simulink model "flatball_6dof"  (R2021b)
settings: Solver=ode1be  StartTime=0.0  StopTime=30  FixedStep=1e-3  MaxStep=0.01  MinStep=0.01  RelTol=1e-3
values from neighbouring files (symbols this model uses):
  amb = evalin( 'base', 'amb')    [flatball_6dof_eqom.m]
  C = evalin( 'base', 'C')    [flatball_6dof_eqom.m]
  disc = evalin( 'base', 'disc')    [flatball_6dof_eqom.m]    (also in flatball_6dof_init.m = struct; flatball_init_disc_params.m = struct)
  X0_z1m_at_rest = [1e-3 1e-3 -1, -1e-6 1e-6 -1e-6, 0 0 1e-6, 0 0 -1e-6]    [flatball_6dof_wrk.m]    (also in hummel_thesis_mdl_validation.m)
undefined symbols (not defined in the file or in its folder): clock, flatball, flatball_6dof_plnt_lib, HandH
libraries: simulink x6, aerolibanim x3, aerolibnav x3, matrix_library x3, mspfiltlib x1, hucker_lib x1
(part 1 of 3)
settings Model: Creator=misc.protolabs@gmail.com  LastModifiedBy=schae
settings SolverCC: InitialStep=0.01  NumberNewtonIterations=10
settings DataIOCC: SaveFormat=StructureWithTime  SaveOutput=off  DSMLogging=off  SaveTime=off  ReturnWorkspaceOutputsName=simout
settings DebuggingCC: InheritedTsInSrcMsg=none

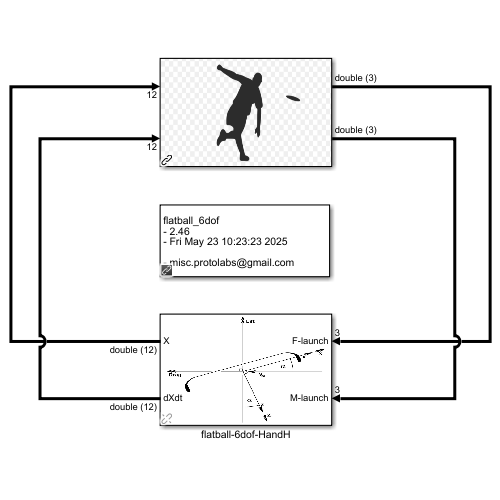
[thumbnail: Simulink's stored preview of the top-level diagram]
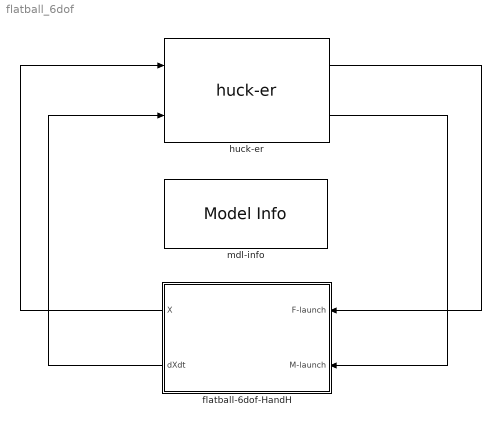
== system flatball_6dof ==
  flatball-6dof-HandH : Subsystem  AncestorBlock=flatball_6dof_plnt_lib/flatball-6dof-HandH
      mask Display: image('C:\.local\desktop\misc.protolabs\flatball-aero-ssl\arxiv\img\screenshots\flatball-6dof.png'); % Use "Edit Image" on toolstrip to change.
  huck-er : hucker_lib/huck-er  SystemSampleTime=-1  VariantActivationTime=update diagram  Latency=0  AutoFrameSizeCalculation=off
      mask Display: image('C:\.local\desktop\misc.protolabs\flatball-aero-ssl\arxiv\img\screenshots\hucker.png'); % Use "Edit Image" on toolstrip to change.
  mdl-info : simulink/Model-Wide Utilities/Model Info  Frame=on  DisplayStringWithTags=|  HorizontalTextAlignment=Left  LeftAlignmentValue=0.02
      | flatball_6dof
      | - %<ModelVersion>
      | - %<LastModificationDate>
      | 
      | - %<Creator>
  wires:
  flatball-6dof-HandH/2(dXdt) -> huck-er/2
  flatball-6dof-HandH/1(X) -> huck-er/1
  huck-er/1 -> flatball-6dof-HandH/1(F-launch)
  huck-er/2 -> flatball-6dof-HandH/2(M-launch)

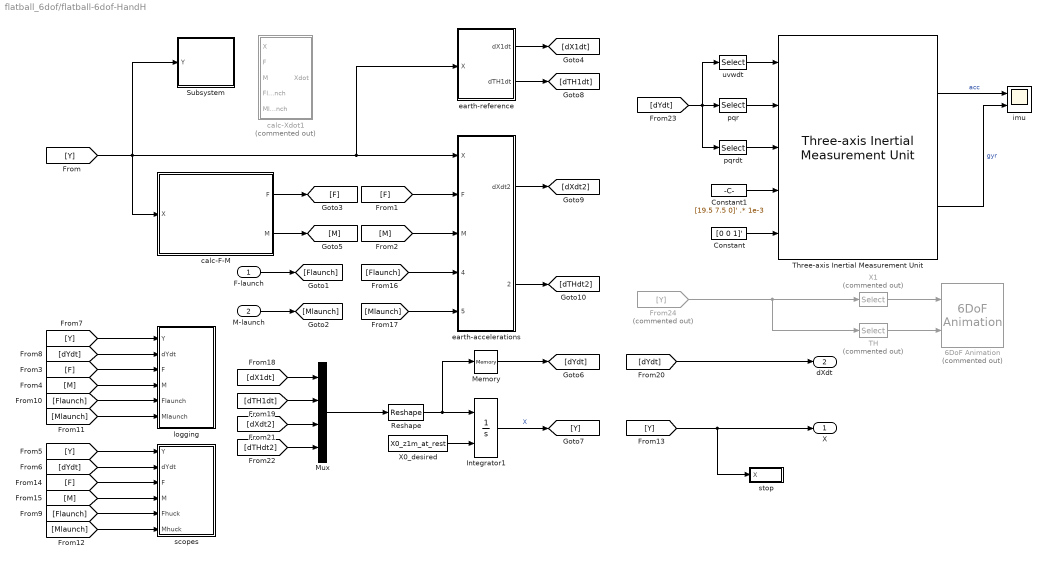
== system flatball_6dof/flatball-6dof-HandH ==
  F-launch : Inport
  M-launch : Inport  Port=2
  6DoF Animation : aerolibanim/6DoF Animation  Commented=on  u1=[0 50 -20 20 -5 0]  u2=0.01  u3=1.0  u4=[50 0 0]  u5=Fixed position  u6=[150 150 25]  u7=10  u8=on
  Constant : Constant  Value=[0 0 1]'
  Constant1 : Constant  Value=[19.5 7.5 0]' .* 1e-3
  From24 : From  Commented=on  GotoTag=Y
  Integrator1 : Integrator  InitialConditionSource=external
  Memory : Memory
  Mux : Mux
  Reshape : Reshape
  Subsystem : Subsystem
  TH : Selector  Commented=on  InputPortWidth=12  IndexOptions=Index vector (dialog)  Indices=[4 5 6]  OutputSizes=1
  Three-axis Inertial Measurement Unit : aerolibnav/Three-axis Inertial Measurement Unit  units=Metric (MKS)  imu=[0 0 0]  i_Ts=0.01  dtype_a=on  w_a=2*pi*50  z_a=0.707  a_sf_cc=[1 0 0; 0 1 0; 0 0 1]  a_bias=[0 0 0]  a_sat=[-1 -1 -1 1 1 1] .* 16*amb.g  dtype_g=on  w_g=2*pi*50  z_g=0.707  g_sf_cc=[1 0 0; 0 1 0; 0 0 1]  g_bias=[0 0 0]  g_sens=[0 0 0]  g_sat=[-1 -1 -1 1 1 1] .* 4000*C.DEG2RAD  i_rand=on  i_seeds=ceil( round( clock, 1))  i_pow=[1 1 1 0.1 0.1 0.1] .* 1e-4
  X0_desired : Constant  Value=X0_z1m_at_rest
  X1 : Selector  Commented=on  InputPortWidth=12  IndexOptions=Index vector (dialog)  Indices=[1 2 3]  OutputSizes=1
  calc-F-M : Subsystem
  calc-Xdot1 : Subsystem  Commented=on
  earth-accelerations : Subsystem
  earth-reference : Subsystem
  imu : Scope  NumInputPorts=2
  logging : Subsystem
  pqr : Selector  InputPortWidth=12  IndexOptions=Index vector (dialog)  Indices=[4 5 6]  OutputSizes=1
  pqrdt : Selector  InputPortWidth=12  IndexOptions=Index vector (dialog)  Indices=[10 11 12]  OutputSizes=1
  scopes : Subsystem
  stop : Subsystem
  uvwdt : Selector  InputPortWidth=12  IndexOptions=Index vector (dialog)  Indices=[7 8 9]  OutputSizes=1
  X : Outport
  dXdt : Outport  Port=2
  wires:
  [Flaunch] -> scopes/5(Fhuck)
  [M] -> scopes/4(M)
  [F] -> scopes/3(F)
  [M] -> logging/4(M)
  [Mlaunch] -> logging/6(Mlaunch)
  [Flaunch] -> logging/5(Flaunch)
  [Mlaunch] -> scopes/6(Mhuck)
  [F] -> logging/3(F)
  [Y] -> scopes/1(Y)
  [dYdt] -> scopes/2(dYdt)
  [dYdt] -> logging/2(dYdt)
  [Y] -> logging/1(Y)
  [Y] -> stop/1(X), X/1
  F-launch/1 -> [Flaunch]
  M-launch/1 -> [Mlaunch]
  [Y] -> earth-reference/1(X), earth-accelerations/1(X), Subsystem/1(Y), calc-F-M/1(X)
  [M] -> earth-accelerations/3(M)
  X0_desired/1 -> Integrator1/2
  [F] -> earth-accelerations/2(F)
  calc-F-M/2(M) -> [M]
  calc-F-M/1(F) -> [F]
  Integrator1/1 -> [Y]  "X"
  [Flaunch] -> earth-accelerations/4(Flaunch)
  [Mlaunch] -> earth-accelerations/5(Mlaunch)
  Memory/1 -> [dYdt]
  earth-reference/1(dX1dt) -> [dX1dt]
  earth-reference/2(dTH1dt) -> [dTH1dt]
  earth-accelerations/1(dXdt2) -> [dXdt2]
  earth-accelerations/2(dTHdt2) -> [dTHdt2]
  [dTHdt2] -> Mux/4
  [dXdt2] -> Mux/3
  [dTH1dt] -> Mux/2
  [dX1dt] -> Mux/1
  Mux/1 -> Reshape/1
  [dYdt] -> dXdt/1
  Reshape/1 -> Memory/1, Integrator1/1
  [dYdt] -> uvwdt/1, pqrdt/1, pqr/1
  pqr/1 -> Three-axis Inertial Measurement Unit/2
  Constant/1 -> Three-axis Inertial Measurement Unit/5
  Constant1/1 -> Three-axis Inertial Measurement Unit/4
  pqrdt/1 -> Three-axis Inertial Measurement Unit/3
  uvwdt/1 -> Three-axis Inertial Measurement Unit/1
  Three-axis Inertial Measurement Unit/1 -> imu/1  "acc"
  Three-axis Inertial Measurement Unit/2 -> imu/2  "gyr"
  From24/1 -> TH/1, X1/1
  TH/1 -> 6DoF Animation/2
  X1/1 -> 6DoF Animation/1

== system flatball_6dof/flatball-6dof-HandH/Subsystem ==
  Y : Inport
  Product : Product  Multiplication=Matrix(*)
  Scope : Scope  NumInputPorts=2
  TH : Selector  InputPortWidth=12  IndexOptions=Index vector (dialog)  Indices=[4 5 6]  OutputSizes=1
  TH1 : Selector  InputPortWidth=3  IndexOptions=Index vector (dialog)  Indices=[1 2]  OutputSizes=1
  TH2 : Selector  InputPortWidth=3  IndexOptions=Index vector (dialog)  Indices=[1 2]  OutputSizes=1
  Terminator : Terminator
  Transpose : Math  Operator=transpose  SaturateOnIntegerOverflow=on
  attitude-transform : MATLAB Function  TreatAsAtomicUnit=on
  rate-transform : MATLAB Function  TreatAsAtomicUnit=on
  wires:
  TH/1 -> Product/2, TH1/1, rate-transform/1(TH), attitude-transform/1(TH)
  rate-transform/1(T) -> [Tr21]
  attitude-transform/1(T) -> [Ta21]
  Y/1 -> TH/1
  [Tr21] -> Terminator/1
  [Ta21] -> Transpose/1
  Transpose/1 -> Product/1
  Product/1 -> TH2/1  "TH2"
  TH1/1 -> Scope/1
  TH2/1 -> Scope/2

== system flatball_6dof/flatball-6dof-HandH/calc-F-M ==
  X : Inport
  From1 : From  Commented=on  GotoTag=X
  From10 : From  Commented=on  GotoTag=F
  From11 : From  Commented=on  GotoTag=M
  From5 : From  Commented=on  GotoTag=alpha
  From6 : From  Commented=on  GotoTag=T
  From9 : From  Commented=on  GotoTag=wD
  TH : Selector  InputPortWidth=12  IndexOptions=Index vector (dialog)  Indices=[4 5 6]  OutputSizes=1
  T_c_N : MATLAB Function  TreatAsAtomicUnit=on
  calc-F : Subsystem
  calc-M : Subsystem
  calc-alpha : Subsystem
  lab : Subsystem  Commented=on
  F : Outport
  M : Outport  Port=2
  wires:
  From1/1 -> lab/1(X)
  From10/1 -> lab/5(F)
  From6/1 -> lab/2(T)
  X/1 -> TH/1, calc-M/1(X), calc-alpha/1(X), calc-F/1(X)
  [T] -> calc-M/2(T_c_N), calc-F/2(T_c_N)
  From9/1 -> lab/3(wD)
  [T] -> calc-alpha/2(T_c_N)
  [alpha] -> calc-F/3(alpha), calc-M/3(alpha)
  From11/1 -> lab/6(M)
  calc-alpha/1(alpha) -> [alpha]
  From5/1 -> lab/4(alpha)
  calc-F/1(F) -> F/1  "F2"
  calc-M/1(M) -> M/1  "M2"
  TH/1 -> T_c_N/1(TH)
  T_c_N/1(T_c_N) -> [T]

== system flatball_6dof/flatball-6dof-HandH/calc-Xdot1 ==
  X : Inport
  F : Inport  Port=2
  M : Inport  Port=3
  Flaunch : Inport  Port=4
  Mlaunch : Inport  Port=5
  Mux{,1..3} (4 alike) : Mux  Inputs=2
  Product1 : Product  Inputs=*/
  Reshape : Reshape
  Reshape1 : Reshape
  Reshape2 : Reshape
  Scope : Scope
  Scope1 : Scope
  Scope2 : Scope
  Selector : Selector  InputPortWidth=12  IndexOptions=Index vector (dialog)  Indices=[1 2 3 7 8 9 4 5 6 10 11 12]  OutputSizes=1
  Sum : Sum  Inputs=2
  calc-THdot : MATLAB Function  TreatAsAtomicUnit=on
  calc-Xdot : MATLAB Function  TreatAsAtomicUnit=on
  dTHdt : Selector  InputPortWidth=12  IndexOptions=Index vector (dialog)  Indices=[10 11 12]  OutputSizes=1
  dXdt : Selector  InputPortWidth=12  IndexOptions=Index vector (dialog)  Indices=[7 8 9]  OutputSizes=1
  mg : Constant  Value=disc.m
  Xdot : Outport
  wires:
  Reshape/1 -> Mux3/2
  Mux2/1 -> Mux/2
  Reshape1/1 -> Mux2/2
  dTHdt/1 -> Mux2/1
  dXdt/1 -> Mux1/1, calc-Xdot/1(dXdt), Mux3/1
  Reshape2/1 -> Sum/1
  Mux1/1 -> Scope/1, Mux/1
  calc-Xdot/1(Xdot) -> Reshape/1  "Xdot"
  calc-THdot/1(dTHdt2) -> Reshape1/1  "THdot"
  Product1/1 -> Mux1/2
  Sum/1 -> Product1/1, Scope2/1
  mg/1 -> Product1/2
  Flaunch/1 -> Sum/2, calc-Xdot/3(Flaunch)
  F/1 -> calc-Xdot/2(F), Reshape2/1
  Mlaunch/1 -> calc-THdot/3(Mlaunch)
  Selector/1 -> Xdot/1
  M/1 -> calc-THdot/2(M)
  X/1 -> calc-THdot/1(X), dXdt/1, dTHdt/1
  Mux/1 -> Selector/1

== system flatball_6dof/flatball-6dof-HandH/earth-accelerations ==
  X : Inport
  F : Inport  Port=2
  M : Inport  Port=3
  Flaunch : Inport  Port=4
  Mlaunch : Inport  Port=5
  Product1 : Product  Inputs=*/
  Sum : Sum  Inputs=2
  Sum1 : Sum  Inputs=2
  calc-THdot : MATLAB Function  TreatAsAtomicUnit=on
  mg : Constant  Value=disc.m
  dXdt2 : Outport
  dTHdt2 : Outport  Port=2
  wires:
  X/1 -> calc-THdot/1(X)
  Flaunch/1 -> Sum/2
  mg/1 -> Product1/2
  Sum/1 -> Product1/1
  Product1/1 -> dXdt2/1
  calc-THdot/1(dTHdt2) -> dTHdt2/1  "THdot"
  F/1 -> Sum/1
  Mlaunch/1 -> Sum1/2
  M/1 -> Sum1/1
  Sum1/1 -> calc-THdot/2(M)

== system flatball_6dof/flatball-6dof-HandH/earth-reference ==
  X : Inport
  dTHdt : Selector  InputPortWidth=12  IndexOptions=Index vector (dialog)  Indices=[10 11 12]  OutputSizes=1
  dXdt : Selector  InputPortWidth=12  IndexOptions=Index vector (dialog)  Indices=[7 8 9]  OutputSizes=1
  dX1dt : Outport
  dTH1dt : Outport  Port=2
  wires:
  X/1 -> dXdt/1, dTHdt/1
  dTHdt/1 -> dTH1dt/1
  dXdt/1 -> dX1dt/1

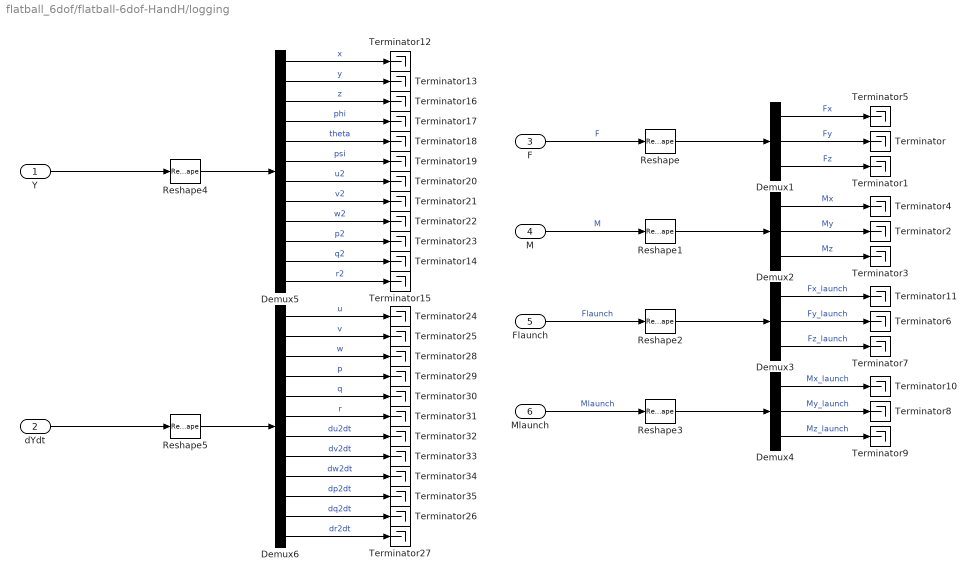
== system flatball_6dof/flatball-6dof-HandH/logging ==
  Y : Inport
  dYdt : Inport  Port=2
  F : Inport  Port=3
  M : Inport  Port=4
  Flaunch : Inport  Port=5
  Mlaunch : Inport  Port=6
  Demux{1..4} (4 alike) : Demux  Outputs=3
  Demux5 : Demux  Outputs=[1 1 1 1 1 1 1 1 1 1 1 1]
  Demux6 : Demux  Outputs=[1 1 1 1 1 1 1 1 1 1 1 1]
  Reshape{,1..5} (6 alike) : Reshape
  Terminator{,1..35} (36 alike) : Terminator
  wires:
  Reshape1/1 -> Demux2/1
  Demux2/3 -> Terminator3/1  "Mz"
  Demux2/1 -> Terminator4/1  "Mx"
  Reshape2/1 -> Demux3/1
  Demux1/3 -> Terminator1/1  "Fz"
  Demux1/2 -> Terminator/1  "Fy"
  Demux2/2 -> Terminator2/1  "My"
  Demux3/3 -> Terminator7/1  "Fz_launch"
  M/1 -> Reshape1/1  "M"
  Demux4/2 -> Terminator8/1  "My_launch"
  Demux1/1 -> Terminator5/1  "Fx"
  Reshape/1 -> Demux1/1
  Demux4/1 -> Terminator10/1  "Mx_launch"
  Demux4/3 -> Terminator9/1  "Mz_launch"
  Reshape3/1 -> Demux4/1
  Flaunch/1 -> Reshape2/1  "Flaunch"
  Demux3/1 -> Terminator11/1  "Fx_launch"
  Demux3/2 -> Terminator6/1  "Fy_launch"
  F/1 -> Reshape/1  "F"
  Mlaunch/1 -> Reshape3/1  "Mlaunch"
  Demux5/3 -> Terminator16/1  "z"
  Demux5/1 -> Terminator12/1  "x"
  Demux5/8 -> Terminator21/1  "v2"
  Demux5/9 -> Terminator22/1  "w2"
  Reshape4/1 -> Demux5/1
  Demux5/2 -> Terminator13/1  "y"
  Demux5/12 -> Terminator15/1  "r2"
  Demux5/10 -> Terminator23/1  "p2"
  Demux5/7 -> Terminator20/1  "u2"
  Demux5/5 -> Terminator18/1  "theta"
  Demux5/6 -> Terminator19/1  "psi"
  Demux5/11 -> Terminator14/1  "q2"
  Demux5/4 -> Terminator17/1  "phi"
  Y/1 -> Reshape4/1
  dYdt/1 -> Reshape5/1
  Demux6/4 -> Terminator29/1  "p"
  Demux6/11 -> Terminator26/1  "dq2dt"
  Demux6/6 -> Terminator31/1  "r"
  Demux6/5 -> Terminator30/1  "q"
  Demux6/7 -> Terminator32/1  "du2dt"
  Demux6/10 -> Terminator35/1  "dp2dt"
  Demux6/12 -> Terminator27/1  "dr2dt"
  Demux6/2 -> Terminator25/1  "v"
  Reshape5/1 -> Demux6/1
  Demux6/9 -> Terminator34/1  "dw2dt"
  Demux6/8 -> Terminator33/1  "dv2dt"
  Demux6/1 -> Terminator24/1  "u"
  Demux6/3 -> Terminator28/1  "w"

== system flatball_6dof/flatball-6dof-HandH/scopes ==
  Y : Inport
  dYdt : Inport  Port=2
  F : Inport  Port=3
  M : Inport  Port=4
  Fhuck : Inport  Port=5
  Mhuck : Inport  Port=6
  Compare To Constant : simulink/Logic and Bit Operations/Compare To Constant  relop=>=  const=0.0  OutDataTypeStr=boolean
  Demux : Demux  Outputs=[3 3 3 3]
  Demux1 : Demux  Outputs=[3 3 3 3]
  Selector : Selector  InputPortWidth=3  IndexOptions=Index vector (dialog)  Indices=[3]  OutputSizes=1
  Selector1 : Selector  InputPortWidth=3  IndexOptions=Index vector (dialog)  Indices=[1 2]  OutputSizes=1
  Stop Simulation : Stop
  Sum1 : Sum
  Sum2 : Sum
  TH1 : Scope
  TH1dot : Scope
  TH2dot : Scope
  TH2dotdot : Scope
  X1 : Scope
  X1dot : Scope
  X2dot : Scope
  X2dotdot : Scope
  eml-6dof : Subsystem  Commented=on
  flatball-F,M : Scope  NumInputPorts=2
  huck-F,M : Scope  NumInputPorts=2
  net-F,M : Scope  NumInputPorts=2
  work-in-progress : Subsystem  Commented=on
  wires:
  Sum2/1 -> net-F,M/2
  Mhuck/1 -> Sum2/2, huck-F,M/2
  Sum1/1 -> net-F,M/1
  Fhuck/1 -> Sum1/2, huck-F,M/1
  F/1 -> Sum1/1, flatball-F,M/1
  M/1 -> Sum2/1, flatball-F,M/2
  Demux/4 -> TH2dot/1
  dYdt/1 -> Demux1/1
  Selector/1 -> Compare To Constant/1
  Demux1/2 -> TH1dot/1
  Demux/2 -> Selector1/1
  Selector1/1 -> TH1/1
  Demux1/1 -> X1dot/1
  Demux/3 -> X2dot/1
  Demux1/4 -> TH2dotdot/1
  Compare To Constant/1 -> Stop Simulation/1
  Y/1 -> Demux/1
  Demux1/3 -> X2dotdot/1
  Demux/1 -> X1/1, Selector/1

== system flatball_6dof/flatball-6dof-HandH/stop ==
  X : Inport
  Compare To Constant : simulink/Logic and Bit Operations/Compare To Constant  relop=>=  const=0  OutDataTypeStr=boolean
  Selector : Selector  InputPortWidth=12  IndexOptions=Index vector (dialog)  Indices=[3]  OutputSizes=1
  Stop Simulation : Stop
  wires:
  Selector/1 -> Compare To Constant/1
  Compare To Constant/1 -> Stop Simulation/1
  X/1 -> Selector/1

== system flatball_6dof/flatball-6dof-HandH/calc-F-M/calc-F ==
  X : Inport
  T_c_N : Inport  Port=2
  alpha : Inport  Port=3
  Fg_N : Constant  Value=[0 0 disc.m*amb.g]'
  Terminator{,1..3} (4 alike) : Terminator
  aero-coeff : Subsystem
  calc-F : MATLAB Function  TreatAsAtomicUnit=on
  dXdt : Selector  InputPortWidth=12  IndexOptions=Index vector (dialog)  Indices=[7 8 9]  OutputSizes=1
  q-inf : Subsystem
  F : Outport
  wires:
  dXdt/1 -> calc-F/1(vel)
  X/1 -> dXdt/1, q-inf/1(X)
  T_c_N/1 -> calc-F/2(T_c_N)
  Fg_N/1 -> calc-F/3(Fg_N)
  calc-F/1(F) -> F/1  "F"
  q-inf/1(q-inf-S) -> calc-F/6(q_inf_times_S)
  alpha/1 -> aero-coeff/1(alpha)
  aero-coeff/1(Cl) -> calc-F/4(CLift)
  aero-coeff/2(Cd) -> calc-F/5(CDrag)
  q-inf/2(q-inf-S-d) -> Terminator/1
  calc-F/2(lift) -> Terminator1/1  "lift"
  calc-F/3(drag) -> Terminator2/1  "drag"
  calc-F/4(vmag) -> Terminator3/1  "v_inf"

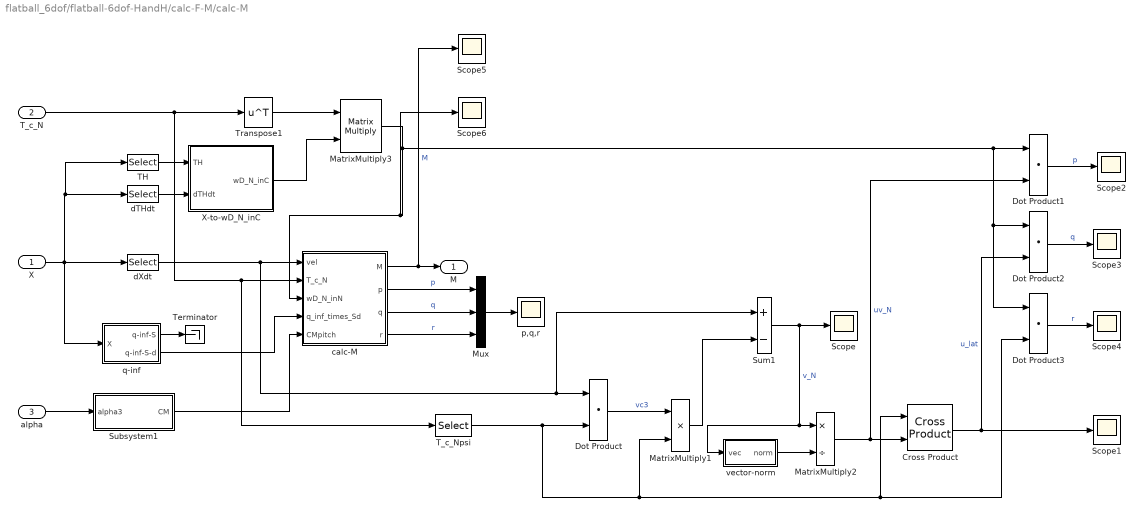
== system flatball_6dof/flatball-6dof-HandH/calc-F-M/calc-M ==
  X : Inport
  T_c_N : Inport  Port=2
  alpha : Inport  Port=3
  Cross Product : matrix_library/Cross Product
      settings: SourceProductBaseCode=SL
  Dot Product{,1..3} (4 alike) : DotProduct  InputSameDT=on  OutDataTypeStr=Inherit: Inherit via internal rule
  MatrixMultiply1 : Product
  MatrixMultiply2 : Product  Inputs=*/
  MatrixMultiply3 : Product  Multiplication=Matrix(*)
  Mux : Mux  Inputs=3
  Scope{,1..6} (7 alike) : Scope
  Subsystem1 : Subsystem
  Sum1 : Sum  Inputs=+-
  TH : Selector  InputPortWidth=12  IndexOptions=Index vector (dialog)  Indices=[4 5 6]  OutputSizes=1
  T_c_Npsi : Selector  NumberOfDimensions=2  InputPortWidth=[3,3]  IndexOptions=Index vector (dialog),Index vector (dialog)  Indices=[1 2 3],[3]  OutputSizes=1,1
  Terminator : Terminator
  Transpose1 : Math  Operator=transpose  SaturateOnIntegerOverflow=on
  X-to-wD_N_inC : MATLAB Function  TreatAsAtomicUnit=on
  calc-M : MATLAB Function  TreatAsAtomicUnit=on
  dTHdt : Selector  InputPortWidth=12  IndexOptions=Index vector (dialog)  Indices=[10 11 12]  OutputSizes=1
  dXdt : Selector  InputPortWidth=12  IndexOptions=Index vector (dialog)  Indices=[7 8 9]  OutputSizes=1
  p,q,r : Scope
  q-inf : Subsystem
  vector-norm : MATLAB Function  TreatAsAtomicUnit=on
  M : Outport
  wires:
  alpha/1 -> Subsystem1/1(alpha3)
  calc-M/1(M) -> Scope5/1, M/1  "M"
  T_c_N/1 -> Transpose1/1, T_c_Npsi/1, calc-M/2(T_c_N)
  X/1 -> TH/1, dTHdt/1, dXdt/1, q-inf/1(X)
  q-inf/2(q-inf-S-d) -> calc-M/4(q_inf_times_Sd)
  Subsystem1/1(CM) -> calc-M/5(CMpitch)
  q-inf/1(q-inf-S) -> Terminator/1
  calc-M/2(p) -> Mux/1  "p"
  calc-M/3(q) -> Mux/2  "q"
  calc-M/4(r) -> Mux/3  "r"
  dXdt/1 -> Sum1/1, Dot Product/1, calc-M/1(vel)
  Mux/1 -> p,q,r/1
  TH/1 -> X-to-wD_N_inC/1(TH)
  dTHdt/1 -> X-to-wD_N_inC/2(dTHdt)
  Transpose1/1 -> MatrixMultiply3/1
  X-to-wD_N_inC/1(wD_N_inC) -> MatrixMultiply3/2
  MatrixMultiply3/1 -> calc-M/3(wD_N_inN), Scope6/1, Dot Product3/1, Dot Product2/1, Dot Product1/1
  T_c_Npsi/1 -> MatrixMultiply1/2, Dot Product3/2, Cross Product/1, Dot Product/2
  Dot Product/1 -> MatrixMultiply1/1  "vc3"
  MatrixMultiply1/1 -> Sum1/2
  Sum1/1 -> vector-norm/1(vec), MatrixMultiply2/1, Scope/1  "v_N"
  vector-norm/1(norm) -> MatrixMultiply2/2
  MatrixMultiply2/1 -> Dot Product1/2, Cross Product/2  "uv_N"
  Cross Product/1 -> Scope1/1, Dot Product2/2  "u_lat"
  Dot Product1/1 -> Scope2/1  "p"
  Dot Product2/1 -> Scope3/1  "q"
  Dot Product3/1 -> Scope4/1  "r"

== system flatball_6dof/flatball-6dof-HandH/calc-F-M/calc-alpha ==
  X : Inport
  T_c_N : Inport  Port=2
  Dot Product : DotProduct  InputSameDT=on  OutDataTypeStr=Inherit: Inherit via internal rule
  MatrixMultiply3 : Product
  Scope : Scope
  Sum : Sum  Inputs=+-
  calc-alpha : MATLAB Function  TreatAsAtomicUnit=on
  calc-alpha1 : MATLAB Function  TreatAsAtomicUnit=on
  dXdt : Selector  InputPortWidth=12  IndexOptions=Index vector (dialog)  Indices=[7 8 9]  OutputSizes=1
  alpha : Outport
  wires:
  calc-alpha/1(alpha) -> alpha/1  "alpha"
  X/1 -> dXdt/1
  T_c_N/1 -> calc-alpha1/1(T_c_N), calc-alpha/2(T_c_N)
  dXdt/1 -> Dot Product/1, Sum/1, calc-alpha/1(dXdt)
  Dot Product/1 -> MatrixMultiply3/1
  MatrixMultiply3/1 -> Sum/2
  Sum/1 -> Scope/1
  calc-alpha1/1(T_c_Npsi) -> MatrixMultiply3/2, Dot Product/2

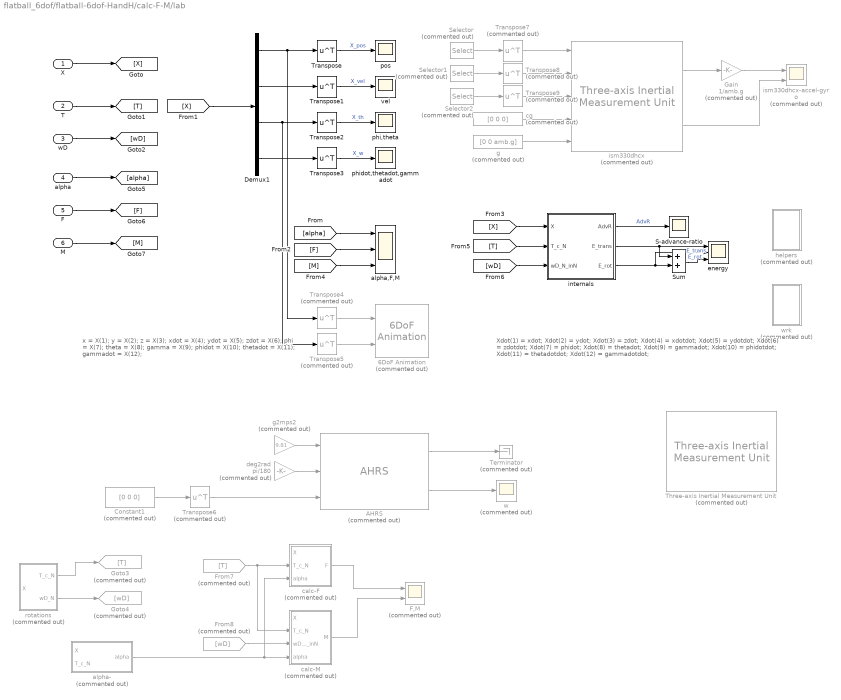
== system flatball_6dof/flatball-6dof-HandH/calc-F-M/lab ==
  note: x = X(1); y = X(2); z = X(3);
      | xdot = X(4); ydot = X(5); zdot = X(6);
      |
      | phi = X(7); theta = X(8); gamma = X(9);
      | phidot = X(10); thetadot = X(11); gammadot = X(12);
  note: Xdot(1) = xdot; Xdot(2) = ydot; Xdot(3) = zdot;
      | Xdot(4) = xdotdot; Xdot(5) = ydotdot; Xdot(6) = zdotdot;
      |
      | Xdot(7) = phidot; Xdot(8) = thetadot; Xdot(9) = gammadot;
      | Xdot(10) = phidotdot; Xdot(11) = thetadotdot; Xdot(12) = gammadotdot;
  X : Inport
  T : Inport  Port=2
  wD : Inport  Port=3
  alpha : Inport  Port=4
  F : Inport  Port=5
  M : Inport  Port=6
  6DoF Animation : aerolibanim/6DoF Animation  Commented=on  u1=[-20 50 -20 50 -20 5]  u2=0.1  u3=1.0  u4=[-1 -1 -1]  u5=Fixed position  u6=[-200 -20 -10]  u7=10  u8=on
  AHRS : mspfiltlib/AHRS  Commented=on
      settings: SourceProductBaseCode=TF,NV
  Constant1 : Constant  Commented=on  Value=[0 0 0]
  Demux1 : Demux  Outputs=[3 3 3 3]
  F,M : Scope  Commented=on  NumInputPorts=2
  From7 : From  Commented=on  GotoTag=T
  From8 : From  Commented=on  GotoTag=wD
  Gain : Gain  Commented=on  Gain=1/amb.g
  Goto3 : Goto  Commented=on  GotoTag=T
  Goto4 : Goto  Commented=on  GotoTag=wD
  S-advance-ratio : Scope
  Selector : Selector  Commented=on  InputPortWidth=12  IndexOptions=Index vector (dialog)  Indices=[4 5 6]  OutputSizes=1
  Selector1 : Selector  Commented=on  InputPortWidth=12  IndexOptions=Index vector (dialog)  Indices=[7 8 9]  OutputSizes=1
  Selector2 : Selector  Commented=on  InputPortWidth=12  IndexOptions=Index vector (dialog)  Indices=[7 8 9]  OutputSizes=1
  Sum : Sum  Inputs=2
  Terminator : Terminator  Commented=on
  Three-axis Inertial Measurement Unit : aerolibnav/Three-axis Inertial Measurement Unit  Commented=on  units=Metric (MKS)  imu=[0 0 0]  i_Ts=0  dtype_a=on  w_a=190  z_a=0.707  a_sf_cc=[1 0 0; 0 1 0; 0 0 1]  a_bias=[0 0 0]  a_sat="[-inf  -inf  -inf  inf inf inf]"  dtype_g=on  w_g=190  z_g=0.707  g_sf_cc=[1 0 0; 0 1 0; 0 0 1]  g_bias=[0 0 0]  g_sens=[0 0 0]  g_sat="[-inf  -inf  -inf  inf inf inf]"  i_rand=on  i_seeds=[23093 23094 23095 23096 23097 23098]  i_pow=[0.001 0.001 0.001 0.0001 0.0001 0.0001]
  Transpose{,1..3} (4 alike) : Math  Operator=transpose  SaturateOnIntegerOverflow=on
  Transpose{4..9} (6 alike) : Math  Commented=on  Operator=transpose  SaturateOnIntegerOverflow=on
  alpha,F,M : Scope  NumInputPorts=3
  alpha- : MATLAB Function  Commented=on  TreatAsAtomicUnit=on
  calc-F : Subsystem  Commented=on
  calc-M : Subsystem  Commented=on
  cg : Constant  Commented=on  Value=[0 0 0]
  deg2rad : Gain  Commented=on  Gain=pi/180
  energy : Scope  NumInputPorts=3
  g : Constant  Commented=on  Value=[0 0 amb.g]
  g2mps2 : Gain  Commented=on  Gain=9.81
  helpers : Subsystem  Commented=on
  internals : MATLAB Function  TreatAsAtomicUnit=on
  ism330dhcx : aerolibnav/Three-axis Inertial Measurement Unit  Commented=on  units=Metric (MKS)  imu=[-2e-3 1e-3 -5e-3]  i_Ts=0  dtype_a=on  w_a=190  z_a=0.707  a_sf_cc=[1 0 0; 0 1 0; 0 0 1]  a_bias=[0 0 0]  a_sat="[-inf  -inf  -inf  inf inf inf]"  dtype_g=on  w_g=190  z_g=0.707  g_sf_cc=[1 0 0; 0 1 0; 0 0 1]  g_bias=[0 0 0]  g_sens=[0 0 0]  g_sat="[-inf  -inf  -inf  inf inf inf]"  i_rand=on  i_seeds=[23093 23094 23095 23096 23097 23098]  i_pow=[0.001 0.001 0.001 0.0001 0.0001 0.0001]
  ism330dhcx-accel-gyro : Scope  Commented=on  NumInputPorts=2
  phi,theta : Scope
  phidot,thetadot,gammadot : Scope
  pos : Scope
  rotations : Subsystem  Commented=on
  vel : Scope
  w : Scope  Commented=on
  wrk : Subsystem  Commented=on
  wires:
  From7/1 -> calc-M/2(T_c_N), calc-F/2(T_c_N)
  alpha-/1(alpha) -> calc-F/3(alpha), calc-M/4(alpha)
  From8/1 -> calc-M/3(wD_N_inN)
  calc-M/1(M) -> F,M/2
  calc-F/1(F) -> F,M/1
  rotations/1(T_c_N) -> Goto3/1
  rotations/2(wD_N) -> Goto4/1
  internals/3(E_rot) -> Sum/2, energy/2  "E_rot"
  [wD] -> internals/3(wD_N_inN)
  internals/1(AdvR) -> S-advance-ratio/1  "AdvR"
  [T] -> internals/2(T_c_N)
  Sum/1 -> energy/3
  [X] -> internals/1(X)
  internals/2(E_trans) -> Sum/1, energy/1  "E_trans"
  Demux1/4 -> Transpose3/1
  Demux1/3 -> Transpose5/1, Transpose2/1
  Demux1/1 -> Transpose4/1, Transpose/1
  Demux1/2 -> Transpose1/1
  [X] -> Demux1/1
  X/1 -> [X]
  T/1 -> [T]
  wD/1 -> [wD]
  F/1 -> [F]
  alpha/1 -> [alpha]
  M/1 -> [M]
  [alpha] -> alpha,F,M/1
  [F] -> alpha,F,M/2
  [M] -> alpha,F,M/3
  Transpose/1 -> pos/1  "X_pos"
  Transpose1/1 -> vel/1  "X_vel"
  Transpose2/1 -> phi,theta/1  "X_th"
  Transpose3/1 -> phidot,thetadot,gammadot/1  "X_w"
  Transpose4/1 -> 6DoF Animation/1
  Transpose5/1 -> 6DoF Animation/2
  Transpose6/1 -> AHRS/3
  Constant1/1 -> Transpose6/1
  AHRS/2 -> w/1
  g2mps2/1 -> AHRS/1
  deg2rad/1 -> AHRS/2
  AHRS/1 -> Terminator/1
  Transpose7/1 -> ism330dhcx/1
  Selector/1 -> Transpose7/1
  g/1 -> ism330dhcx/5
  Transpose8/1 -> ism330dhcx/2
  cg/1 -> ism330dhcx/4
  ism330dhcx/1 -> Gain/1
  Transpose9/1 -> ism330dhcx/3
  Selector1/1 -> Transpose8/1
  Selector2/1 -> Transpose9/1
  Gain/1 -> ism330dhcx-accel-gyro/1
  ism330dhcx/2 -> ism330dhcx-accel-gyro/2

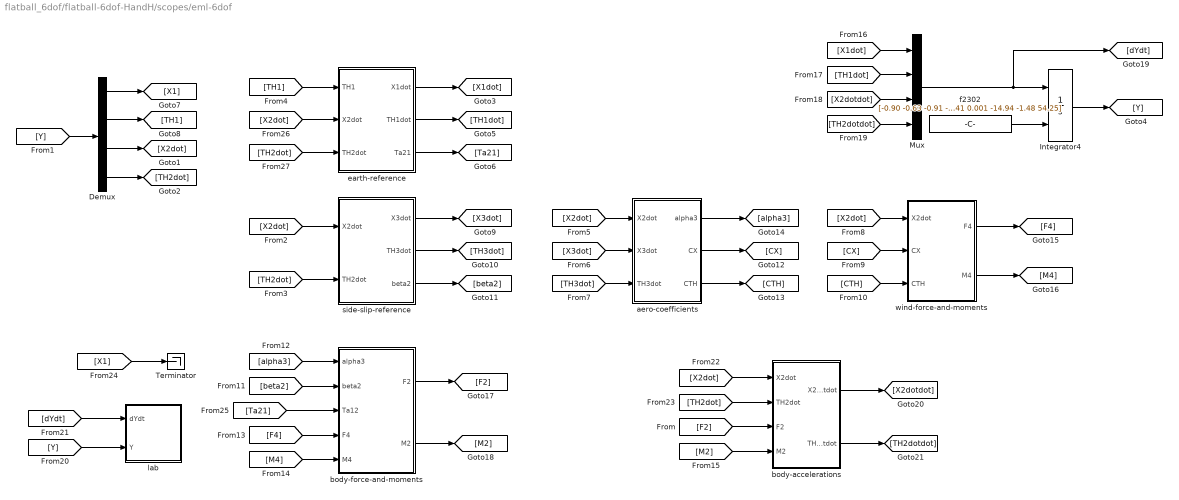
== system flatball_6dof/flatball-6dof-HandH/scopes/eml-6dof ==
  Demux : Demux  Outputs=[3 3 3 3]
  Integrator4 : Integrator  InitialConditionSource=external
  Mux : Mux
  Terminator : Terminator
  aero-coefficients : MATLAB Function  TreatAsAtomicUnit=on
  body-accelerations : MATLAB Function  TreatAsAtomicUnit=on
  body-force-and-moments : MATLAB Function  TreatAsAtomicUnit=on
  earth-reference : MATLAB Function  TreatAsAtomicUnit=on
  f2302 : Constant  Value=[-0.90 -0.63 -0.91 -0.07 0.21 5.03 13.42 -0.41 0.001 -14.94 -1.48 54.25]
  lab : Subsystem
  side-slip-reference : MATLAB Function  TreatAsAtomicUnit=on
  wind-force-and-moments : MATLAB Function  TreatAsAtomicUnit=on
  wires:
  [TH2dot] -> earth-reference/3(TH2dot)
  [X2dot] -> earth-reference/2(X2dot)
  [X1] -> Terminator/1
  [Ta21] -> body-force-and-moments/3(Ta12)
  body-accelerations/1(X2dotdot) -> [X2dotdot]
  body-accelerations/2(TH2dotdot) -> [TH2dotdot]
  [TH2dot] -> body-accelerations/2(TH2dot)
  [X2dot] -> body-accelerations/1(X2dot)
  [M2] -> body-accelerations/4(M2)
  [F2] -> body-accelerations/3(F2)
  [Y] -> lab/2(Y)
  [dYdt] -> lab/1(dYdt)
  Integrator4/1 -> [Y]
  [X2dotdot] -> Mux/3
  f2302/1 -> Integrator4/2
  [X1dot] -> Mux/1
  [TH1dot] -> Mux/2
  Mux/1 -> [dYdt], Integrator4/1
  [TH2dotdot] -> Mux/4
  body-force-and-moments/2(M2) -> [M2]
  body-force-and-moments/1(F2) -> [F2]
  [M4] -> body-force-and-moments/5(M4)
  [F4] -> body-force-and-moments/4(F4)
  wind-force-and-moments/2(M4) -> [M4]
  wind-force-and-moments/1(F4) -> [F4]
  [alpha3] -> body-force-and-moments/1(alpha3)
  [beta2] -> body-force-and-moments/2(beta2)
  [CTH] -> wind-force-and-moments/3(CTH)
  [CX] -> wind-force-and-moments/2(CX)
  [X2dot] -> wind-force-and-moments/1(X2dot)
  aero-coefficients/1(alpha3) -> [alpha3]
  aero-coefficients/2(CX) -> [CX]
  aero-coefficients/3(CTH) -> [CTH]
  [TH3dot] -> aero-coefficients/3(TH3dot)
  [X3dot] -> aero-coefficients/2(X3dot)
  [X2dot] -> aero-coefficients/1(X2dot)
  [TH1] -> earth-reference/1(TH1)
  side-slip-reference/3(beta2) -> [beta2]
  side-slip-reference/2(TH3dot) -> [TH3dot]
  side-slip-reference/1(X3dot) -> [X3dot]
  [TH2dot] -> side-slip-reference/2(TH2dot)
  [X2dot] -> side-slip-reference/1(X2dot)
  Demux/4 -> [TH2dot]
  Demux/3 -> [X2dot]
  Demux/2 -> [TH1]
  Demux/1 -> [X1]
  [Y] -> Demux/1
  earth-reference/3(Ta21) -> [Ta21]
  earth-reference/2(TH1dot) -> [TH1dot]
  earth-reference/1(X1dot) -> [X1dot]

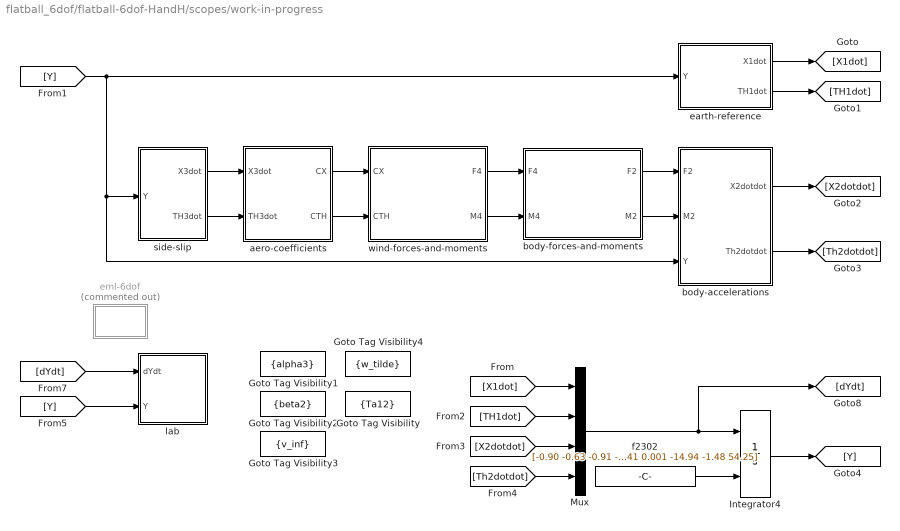
== system flatball_6dof/flatball-6dof-HandH/scopes/work-in-progress ==
  Goto Tag Visibility : GotoTagVisibility  GotoTag=Ta12
  Goto Tag Visibility1 : GotoTagVisibility  GotoTag=alpha3
  Goto Tag Visibility2 : GotoTagVisibility  GotoTag=beta2
  Goto Tag Visibility3 : GotoTagVisibility  GotoTag=v_inf
  Goto Tag Visibility4 : GotoTagVisibility  GotoTag=w_tilde
  Integrator4 : Integrator  InitialConditionSource=external
  Mux : Mux
  aero-coefficients : Subsystem
  body-accelerations : Subsystem
  body-forces-and-moments : Subsystem
  earth-reference : Subsystem
  eml-6dof : Subsystem  Commented=on
  f2302 : Constant  Value=[-0.90 -0.63 -0.91 -0.07 0.21 5.03 13.42 -0.41 0.001 -14.94 -1.48 54.25]
  lab : Subsystem
  side-slip : Subsystem
  wind-forces-and-moments : Subsystem
  wires:
  aero-coefficients/2(CTH) -> wind-forces-and-moments/2(CTH)
  side-slip/1(X3dot) -> aero-coefficients/1(X3dot)
  aero-coefficients/1(CX) -> wind-forces-and-moments/1(CX)
  body-forces-and-moments/1(F2) -> body-accelerations/1(F2)
  side-slip/2(TH3dot) -> aero-coefficients/2(TH3dot)
  wind-forces-and-moments/1(F4) -> body-forces-and-moments/1(F4)
  wind-forces-and-moments/2(M4) -> body-forces-and-moments/2(M4)
  body-forces-and-moments/2(M2) -> body-accelerations/2(M2)
  earth-reference/1(X1dot) -> [X1dot]
  earth-reference/2(TH1dot) -> [TH1dot]
  body-accelerations/2(Th2dotdot) -> [Th2dotdot]
  f2302/1 -> Integrator4/2
  [Y] -> body-accelerations/3(Y), side-slip/1(Y), earth-reference/1(Y)
  Integrator4/1 -> [Y]
  Mux/1 -> Integrator4/1, [dYdt]
  body-accelerations/1(X2dotdot) -> [X2dotdot]
  [TH1dot] -> Mux/2
  [dYdt] -> lab/1(dYdt)
  [Th2dotdot] -> Mux/4
  [X2dotdot] -> Mux/3
  [Y] -> lab/2(Y)
  [X1dot] -> Mux/1

== system flatball_6dof/flatball-6dof-HandH/calc-F-M/calc-F/aero-coeff ==
  alpha : Inport
  Subsystem : Subsystem
  Subsystem1 : Subsystem
  calc-Cd : Subsystem  Commented=on
  calc-Cl : Subsystem  Commented=on
  Cl : Outport
  Cd : Outport  Port=2
  wires:
  alpha/1 -> Subsystem1/1(alpha3), Subsystem/1(alpha3)
  Subsystem1/1(Clift) -> Cl/1  "Clift"
  Subsystem/1(Cdrag) -> Cd/1  "Cdrag"

== system flatball_6dof/flatball-6dof-HandH/calc-F-M/calc-F/q-inf ==
  X : Inport
  Gain : Gain  Gain=0.5
  Product1 : Product  Inputs=3
  Product2 : Product
  S : Constant  Value=disc.A
  Square : Math  Operator=square  SaturateOnIntegerOverflow=on
  d : Constant  Value=disc.d
  dXdt : Selector  InputPortWidth=12  IndexOptions=Index vector (dialog)  Indices=[7 8 9]  OutputSizes=1
  rho : Constant  Value=amb.rho
  vector-norm : MATLAB Function  TreatAsAtomicUnit=on
  q-inf-S : Outport
  q-inf-S-d : Outport  Port=2
  wires:
  Product1/1 -> Gain/1
  rho/1 -> Product1/3
  vector-norm/1(norm) -> Square/1
  S/1 -> Product1/2
  Square/1 -> Product1/1
  Gain/1 -> Product2/1, q-inf-S/1
  X/1 -> dXdt/1
  Product2/1 -> q-inf-S-d/1
  d/1 -> Product2/2
  dXdt/1 -> vector-norm/1(vec)

== system flatball_6dof/flatball-6dof-HandH/calc-F-M/calc-M/Subsystem1 ==
  alpha3 : Inport
  1-D Lookup Table : Lookup_n-D  NumberOfTableDimensions=1  BreakpointsForDimension1=disc.aoa_data  Table=disc.CM_data  InterpMethod=Cubic spline  ExtrapMethod=Cubic spline  InternalRulePriority=Speed  RndMeth=Simplest  InputSameDT=on
  Ground : Ground
  Product1 : Product  Inputs=**
  Sum1 : Sum
  Sum2 : Sum
  Terminator : Terminator
  mg : Constant  Value=disc.CM0
  mg1 : Constant  Value=disc.CMa
  CM : Outport
  wires:
  mg1/1 -> Product1/2
  alpha3/1 -> 1-D Lookup Table/1, Product1/1
  Product1/1 -> Sum2/2
  1-D Lookup Table/1 -> Sum1/1
  mg/1 -> Sum2/1
  Sum2/1 -> Terminator/1
  Sum1/1 -> CM/1
  Ground/1 -> Sum1/2

== system flatball_6dof/flatball-6dof-HandH/calc-F-M/calc-M/q-inf ==
  X : Inport
  Gain : Gain  Gain=0.5
  Product1 : Product  Inputs=3
  Product2 : Product
  S : Constant  Value=disc.A
  Square : Math  Operator=square  SaturateOnIntegerOverflow=on
  d : Constant  Value=disc.d
  dXdt : Selector  InputPortWidth=12  IndexOptions=Index vector (dialog)  Indices=[7 8 9]  OutputSizes=1
  rho : Constant  Value=amb.rho
  vector-norm : MATLAB Function  TreatAsAtomicUnit=on
  q-inf-S : Outport
  q-inf-S-d : Outport  Port=2
  wires:
  d/1 -> Product2/2
  Product2/1 -> q-inf-S-d/1
  X/1 -> dXdt/1
  Gain/1 -> q-inf-S/1, Product2/1
  Square/1 -> Product1/1
  S/1 -> Product1/2
  vector-norm/1(norm) -> Square/1
  rho/1 -> Product1/3
  Product1/1 -> Gain/1
  dXdt/1 -> vector-norm/1(vec)

== system flatball_6dof/flatball-6dof-HandH/calc-F-M/lab/calc-F ==
  X : Inport
  T_c_N : Inport  Port=2
  alpha : Inport  Port=3
  Fg_N : Constant  Value=[0 0 disc.m*amb.g]'
  Terminator : Terminator
  X-to-vel : MATLAB Function  TreatAsAtomicUnit=on
  aero-coeff : Subsystem
  calc-F : MATLAB Function  TreatAsAtomicUnit=on
  q-inf : Subsystem
  F : Outport
  wires:
  X-to-vel/1(vel) -> calc-F/1(vel)
  X/1 -> q-inf/1(X), X-to-vel/1(X)
  T_c_N/1 -> calc-F/2(T_c_N)
  Fg_N/1 -> calc-F/3(Fg_N)
  calc-F/1(F) -> F/1
  q-inf/1(q-inf-S) -> calc-F/6(q_inf_times_S)
  alpha/1 -> aero-coeff/1(alpha)
  aero-coeff/1(Cl) -> calc-F/4(CLift)
  aero-coeff/2(Cd) -> calc-F/5(CDrag)
  q-inf/2(q-inf-S-d) -> Terminator/1

== system flatball_6dof/flatball-6dof-HandH/calc-F-M/lab/calc-M ==
  X : Inport
  T_c_N : Inport  Port=2
  wD_N_inN : Inport  Port=3
  alpha : Inport  Port=4
  Terminator : Terminator
  X-to-vel : MATLAB Function  TreatAsAtomicUnit=on
  aero-coeff : Subsystem
  calc-M : MATLAB Function  TreatAsAtomicUnit=on
  q-inf : Subsystem
  M : Outport
  wires:
  alpha/1 -> aero-coeff/1(alpha)
  calc-M/1(M) -> M/1
  T_c_N/1 -> calc-M/2(T_c_N)
  X/1 -> X-to-vel/1(X), q-inf/1(X)
  X-to-vel/1(vel) -> calc-M/1(vel)
  q-inf/2(q-inf-S-d) -> calc-M/5(q_inf_times_Sd)
  aero-coeff/1(Cm) -> calc-M/4(CMpitch)
  wD_N_inN/1 -> calc-M/3(wD_N_inN)
  q-inf/1(q-inf-S) -> Terminator/1

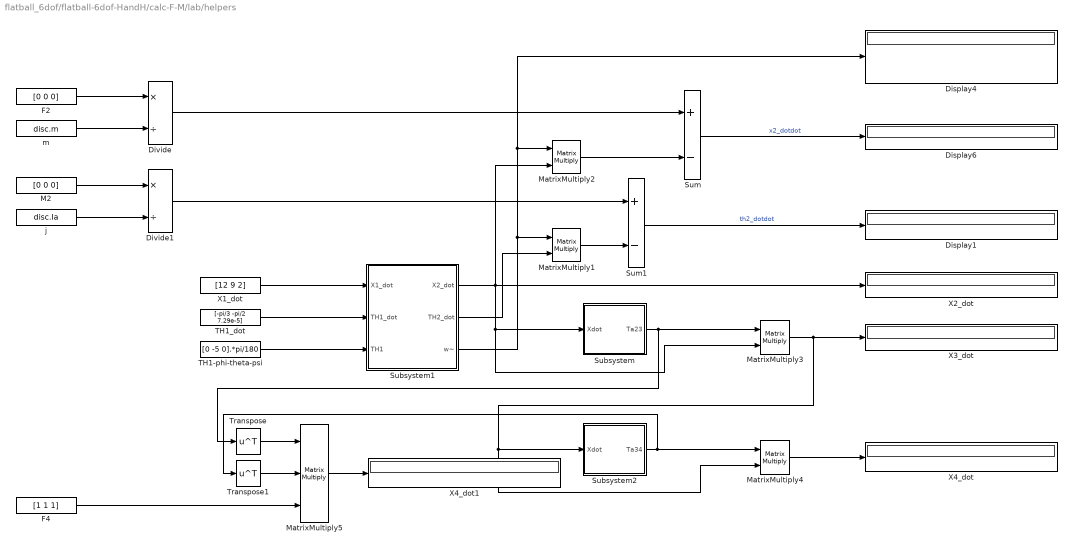
== system flatball_6dof/flatball-6dof-HandH/calc-F-M/lab/helpers ==
  Display1 : Display
  Display4 : Display
  Display6 : Display
  Divide : Product  Inputs=*/
  Divide1 : Product  Inputs=*/
  F2 : Constant  Value=[0 0 0]
  F4 : Constant  Value=[1 1 1]
  M2 : Constant  Value=[0 0 0]
  MatrixMultiply{1..4} (4 alike) : Product  Multiplication=Matrix(*)
  MatrixMultiply5 : Product  Inputs=***  Multiplication=Matrix(*)
  Subsystem : Subsystem
  Subsystem1 : Subsystem
  Subsystem2 : Subsystem
  Sum : Sum  Inputs=+-
  Sum1 : Sum  Inputs=+-
  TH1-phi-theta-psi : Constant  Value=[0 -5 0].*pi/180
  TH1_dot : Constant  Value=[-pi/3 -pi/2 7.29e-5]
  Transpose : Math  Operator=transpose  SaturateOnIntegerOverflow=on
  Transpose1 : Math  Operator=transpose  SaturateOnIntegerOverflow=on
  X1_dot : Constant  Value=[12 9 2]
  X2_dot : Display
  X3_dot : Display
  X4_dot : Display
  X4_dot1 : Display
  j : Constant  Value=disc.Ia
  m : Constant  Value=disc.m
  wires:
  X1_dot/1 -> Subsystem1/1(X1_dot)
  TH1_dot/1 -> Subsystem1/2(TH1_dot)
  TH1-phi-theta-psi/1 -> Subsystem1/3(TH1)
  MatrixMultiply2/1 -> Sum/2
  Subsystem1/3(w~) -> MatrixMultiply1/1, Display4/1, MatrixMultiply2/1
  Subsystem1/1(X2_dot) -> MatrixMultiply2/2, X2_dot/1, MatrixMultiply3/2, Subsystem/1(Xdot)
  F2/1 -> Divide/1
  m/1 -> Divide/2
  Divide/1 -> Sum/1
  Sum/1 -> Display6/1  "x2_dotdot"
  j/1 -> Divide1/2
  M2/1 -> Divide1/1
  Divide1/1 -> Sum1/1
  MatrixMultiply1/1 -> Sum1/2
  Subsystem1/2(TH2_dot) -> MatrixMultiply1/2
  Sum1/1 -> Display1/1  "th2_dotdot"
  Subsystem/1(Ta23) -> Transpose/1, MatrixMultiply3/1
  MatrixMultiply3/1 -> MatrixMultiply4/2, Subsystem2/1(Xdot), X3_dot/1
  Subsystem2/1(Ta34) -> Transpose1/1, MatrixMultiply4/1
  MatrixMultiply4/1 -> X4_dot/1
  Transpose1/1 -> MatrixMultiply5/2
  Transpose/1 -> MatrixMultiply5/1
  F4/1 -> MatrixMultiply5/3
  MatrixMultiply5/1 -> X4_dot1/1

== system flatball_6dof/flatball-6dof-HandH/calc-F-M/lab/rotations ==
  X : Inport
  MatrixMultiply3 : Product  Multiplication=Matrix(*)
  Transpose : Math  Operator=transpose  SaturateOnIntegerOverflow=on
  Transpose1 : Math  Operator=transpose  SaturateOnIntegerOverflow=on
  X-to-T_c_N : MATLAB Function  TreatAsAtomicUnit=on
  X-to-wD_N_inC : MATLAB Function  TreatAsAtomicUnit=on
  T_c_N : Outport
  wD_N : Outport  Port=2
  wires:
  X-to-T_c_N/1(T_c_N) -> Transpose1/1, T_c_N/1
  Transpose1/1 -> MatrixMultiply3/1
  X-to-wD_N_inC/1(wD_N_inC) -> Transpose/1
  Transpose/1 -> MatrixMultiply3/2
  MatrixMultiply3/1 -> wD_N/1
  X/1 -> X-to-wD_N_inC/1(X), X-to-T_c_N/1(X)

== system flatball_6dof/flatball-6dof-HandH/calc-F-M/lab/wrk ==
  6DoF Animation : aerolibanim/6DoF Animation  Commented=on  u1=[-10 100 -20 100 -10 10]  u2=0.01  u3=5  u4=[1 0 -5]  u5=Fixed position  u6=[100 50 -500]  u7=10  u8=on
  Demux : Demux  Commented=on  Outputs=[3 3 3 3]
  From : From  Commented=on  GotoTag=x1
  From1 : From  Commented=on  GotoTag=x1dt
  From2 : From  Commented=on  GotoTag=theta1
  From3 : From  Commented=on  GotoTag=theta1dt
  From5 : From  Commented=on  GotoTag=theta1
  From6 : From  Commented=on  GotoTag=theta1dt
  From7 : From  Commented=on  GotoTag=x1dt
  Transpose{3..6} (4 alike) : Math  Commented=on  Operator=transpose  SaturateOnIntegerOverflow=on
  c&p : Subsystem  Commented=on
  flatball_6dof : MATLAB Function  Commented=on  TreatAsAtomicUnit=on
  flatball_6dof_v1p0 : MATLAB Function  Commented=on  TreatAsAtomicUnit=on
  flatball_6dof_v1p1 : MATLAB Function  Commented=on  TreatAsAtomicUnit=on
  hummel : Subsystem  Commented=on
  wires:
  From/1 -> Transpose3/1
  From2/1 -> Transpose5/1
  From3/1 -> Transpose6/1
  Demux/3 -> 6DoF Animation/2
  Transpose3/1 -> c&p/1(x1)
  Demux/1 -> 6DoF Animation/1
  From1/1 -> Transpose4/1
  Transpose5/1 -> c&p/3(theta1)
  Transpose4/1 -> c&p/2(x1dt)
  Transpose6/1 -> c&p/4(theta1dt)
  From5/1 -> hummel/2(TH)
  From6/1 -> hummel/3(TH-dt)
  From7/1 -> hummel/1(vel)

== system flatball_6dof/flatball-6dof-HandH/scopes/eml-6dof/lab ==
  dYdt : Inport
  Y : Inport  Port=2
  Compare To Constant : simulink/Logic and Bit Operations/Compare To Constant  relop=>=  const=0.0  OutDataTypeStr=boolean
  Demux : Demux  Outputs=[3 3 3 3]
  Demux1 : Demux  Outputs=[3 3 3 3]
  Selector : Selector  InputPortWidth=3  IndexOptions=Index vector (dialog)  Indices=[3]  OutputSizes=1
  Selector1 : Selector  InputPortWidth=3  IndexOptions=Index vector (dialog)  Indices=[1 2]  OutputSizes=1
  Stop Simulation : Stop
  TH1 : Scope
  TH1dot : Scope
  TH2dot : Scope
  TH2dotdot : Scope
  X1 : Scope
  X1dot : Scope
  X2dot : Scope
  X2dotdot : Scope
  wires:
  Demux1/3 -> X2dotdot/1
  Demux1/4 -> TH2dotdot/1
  Demux1/2 -> TH1dot/1
  Demux1/1 -> X1dot/1
  dYdt/1 -> Demux1/1
  Demux/4 -> TH2dot/1
  Demux/3 -> X2dot/1
  Demux/2 -> Selector1/1
  Demux/1 -> X1/1, Selector/1
  Y/1 -> Demux/1
  Selector1/1 -> TH1/1
  Selector/1 -> Compare To Constant/1
  Compare To Constant/1 -> Stop Simulation/1

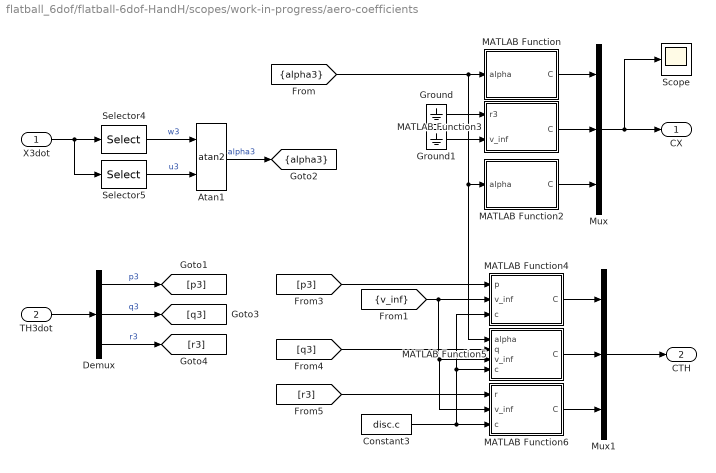
== system flatball_6dof/flatball-6dof-HandH/scopes/work-in-progress/aero-coefficients ==
  X3dot : Inport
  TH3dot : Inport  Port=2
  Atan1 : Trigonometry  Operator=atan2
  Constant3 : Constant  Value=disc.c
  Demux : Demux  Outputs=3
  Ground : Ground
  Ground1 : Ground
  MATLAB Function : MATLAB Function  TreatAsAtomicUnit=on
  MATLAB Function2 : MATLAB Function  TreatAsAtomicUnit=on
  MATLAB Function3 : MATLAB Function  TreatAsAtomicUnit=on
  MATLAB Function4 : MATLAB Function  TreatAsAtomicUnit=on
  MATLAB Function5 : MATLAB Function  TreatAsAtomicUnit=on
  MATLAB Function6 : MATLAB Function  TreatAsAtomicUnit=on
  Mux : Mux  Inputs=3
  Mux1 : Mux  Inputs=3
  Scope : Scope
  Selector4 : Selector  InputPortWidth=3  IndexOptions=Index vector (dialog)  Indices=[3]  OutputSizes=1
  Selector5 : Selector  InputPortWidth=3  IndexOptions=Index vector (dialog)  Indices=[1]  OutputSizes=1
  CX : Outport
  CTH : Outport  Port=2
  tag scope: alpha3=scoped
  wires:
  Selector5/1 -> Atan1/2  "u3"
  Selector4/1 -> Atan1/1  "w3"
  Atan1/1 -> [alpha3]  "alpha3"
  Demux/1 -> [p3]  "p3"
  Demux/2 -> [q3]  "q3"
  Demux/3 -> [r3]  "r3"
  X3dot/1 -> Selector5/1, Selector4/1
  MATLAB Function3/1(C) -> Mux/2
  MATLAB Function2/1(C) -> Mux/3
  MATLAB Function/1(C) -> Mux/1
  MATLAB Function6/1(C) -> Mux1/3
  MATLAB Function5/1(C) -> Mux1/2
  MATLAB Function4/1(C) -> Mux1/1
  Mux/1 -> Scope/1, CX/1
  Mux1/1 -> CTH/1
  [alpha3] -> MATLAB Function2/1(alpha), MATLAB Function5/1(alpha), MATLAB Function/1(alpha)
  Constant3/1 -> MATLAB Function4/3(c), MATLAB Function5/4(c), MATLAB Function6/3(c)
  [v_inf] -> MATLAB Function6/2(v_inf), MATLAB Function5/3(v_inf), MATLAB Function4/2(v_inf)
  [p3] -> MATLAB Function4/1(p)
  [q3] -> MATLAB Function5/2(q)
  [r3] -> MATLAB Function6/1(r)
  TH3dot/1 -> Demux/1
  Ground/1 -> MATLAB Function3/1(r3)
  Ground1/1 -> MATLAB Function3/2(v_inf)

== system flatball_6dof/flatball-6dof-HandH/scopes/work-in-progress/body-accelerations ==
  F2 : Inport
  M2 : Inport  Port=2
  Y : Inport  Port=3
  Constant1 : Constant  Value=disc.I
  Constant2 : Constant  Value=disc.m
  Constant3 : Constant  Value=disc.I ^ -1
  Product : Product  Multiplication=Matrix(*)
  Product1 : Product  Inputs=*/
  Product4 : Product  Inputs=3  Multiplication=Matrix(*)
  Product5 : Product  Multiplication=Matrix(*)
  Sum : Sum  Inputs=+-
  Sum1 : Sum  Inputs=+-
  TH2dot : Selector  InputPortWidth=12  IndexOptions=Index vector (dialog)  Indices=[10 11 12]  OutputSizes=1
  X2dot : Selector  InputPortWidth=12  IndexOptions=Index vector (dialog)  Indices=[7 8 9]  OutputSizes=1
  X2dotdot : Outport
  Th2dotdot : Outport  Port=2
  wires:
  X2dot/1 -> Product/2
  F2/1 -> Product1/1
  Constant2/1 -> Product1/2
  Product1/1 -> Sum/1
  Product/1 -> Sum/2
  Sum/1 -> X2dotdot/1
  M2/1 -> Sum1/1
  Product4/1 -> Sum1/2
  Sum1/1 -> Product5/2
  Constant3/1 -> Product5/1
  Product5/1 -> Th2dotdot/1
  Y/1 -> X2dot/1, TH2dot/1
  [w_tilde] -> Product/1
  [w_tilde] -> Product4/1
  Constant1/1 -> Product4/2
  TH2dot/1 -> Product4/3

== system flatball_6dof/flatball-6dof-HandH/scopes/work-in-progress/body-forces-and-moments ==
  F4 : Inport
  M4 : Inport  Port=2
  Ground{,1..3} (4 alike) : Ground
  Mux : Mux  Inputs=3
  Mux1 : Mux  Inputs=3
  Product{,1..3} (4 alike) : Product  Multiplication=Matrix(*)
  Sum : Sum
  Transpose : Math  Operator=transpose  SaturateOnIntegerOverflow=on
  attitude-transformation : MATLAB Function  TreatAsAtomicUnit=on
  attitude-transformation1 : MATLAB Function  TreatAsAtomicUnit=on
  mg : Subsystem
  F2 : Outport
  M2 : Outport  Port=2
  wires:
  Ground1/1 -> Mux/3
  Ground/1 -> Mux/1
  Mux/1 -> attitude-transformation/1(TH)
  Mux1/1 -> attitude-transformation1/1(TH)
  Ground3/1 -> Mux1/2
  Ground2/1 -> Mux1/1
  attitude-transformation1/1(T) -> Product/2  "Ta32"
  Transpose/1 -> Product/1  "Ta43"
  attitude-transformation/1(T) -> Transpose/1  "Ta34"
  Product/1 -> [Ta42]  "Ta42"
  [Ta42] -> Product1/1
  F4/1 -> Product1/2
  M4/1 -> Product2/2
  [Ta42] -> Product2/1
  Product1/1 -> Sum/1  "F2aero"
  Product2/1 -> M2/1
  Product3/1 -> Sum/2
  Sum/1 -> F2/1
  mg/1(mg) -> Product3/2
  [beta2] -> Mux1/3
  [alpha3] -> Mux/2
  [Ta12] -> Product3/1

== system flatball_6dof/flatball-6dof-HandH/scopes/work-in-progress/earth-reference ==
  Y : Inport
  Product : Product  Multiplication=Matrix(*)
  Product1 : Product  Multiplication=Matrix(*)
  TH1 : Selector  InputPortWidth=12  IndexOptions=Index vector (dialog)  Indices=[4 5 6]  OutputSizes=1
  TH2dot : Selector  InputPortWidth=12  IndexOptions=Index vector (dialog)  Indices=[10 11 12]  OutputSizes=1
  Transpose : Math  Operator=transpose  SaturateOnIntegerOverflow=on
  X2dot : Selector  InputPortWidth=12  IndexOptions=Index vector (dialog)  Indices=[7 8 9]  OutputSizes=1
  attitude-transformation : MATLAB Function  TreatAsAtomicUnit=on
  beta2 : Subsystem
  rate-transformation : MATLAB Function  TreatAsAtomicUnit=on
  v_inf : Subsystem
  w_tilde : Subsystem
  X1dot : Outport
  TH1dot : Outport  Port=2
  tag scope: Ta12=scoped
  wires:
  TH1/1 -> attitude-transformation/1(TH), rate-transformation/1(TH)  "TH1"
  attitude-transformation/1(T) -> [Ta21]
  Y/1 -> TH1/1, X2dot/1, TH2dot/1
  rate-transformation/1(T) -> [Tr21]
  [Ta21] -> Product/1
  X2dot/1 -> Product/2, w_tilde/1(X2dot), v_inf/1(X2dot), beta2/1(X2dot)  "X2dot"
  TH2dot/1 -> Product1/2  "TH2dot"
  [Tr21] -> Product1/1
  Product/1 -> X1dot/1
  Product1/1 -> TH1dot/1
  [Ta21] -> Transpose/1
  Transpose/1 -> [Ta12]

== system flatball_6dof/flatball-6dof-HandH/scopes/work-in-progress/eml-6dof ==
  Integrator4 : Integrator  InitialConditionSource=external
  MATLAB Function : MATLAB Function  TreatAsAtomicUnit=on
  f2302 : Constant  Value=[-0.90 -0.63 -0.91 -0.07 0.21 5.03 13.42 -0.41 0.001 -14.94 -1.48 54.25]
  lab : Subsystem
  wires:
  MATLAB Function/7(X3dot) -> lab/7(X3-dot)
  MATLAB Function/3(X1dot) -> lab/3(X1-dot)
  MATLAB Function/10(beta2) -> lab/10(beta2)
  MATLAB Function/4(TH1dot) -> lab/4(TH1-dot)
  MATLAB Function/6(TH2dot) -> lab/6(TH2-dot)
  MATLAB Function/5(X2dot) -> lab/5(X2-dot)
  MATLAB Function/2(TH1) -> lab/2(TH1)
  [X] -> MATLAB Function/1(X)
  f2302/1 -> MATLAB Function/2(X0), Integrator4/2
  MATLAB Function/1(X1) -> lab/1(X1)
  Integrator4/1 -> [X]  "X"
  MATLAB Function/8(TH3dot) -> lab/8(TH3-dot)
  MATLAB Function/9(alpha3) -> lab/9(alpha3)
  MATLAB Function/11(dydt) -> Integrator4/1

== system flatball_6dof/flatball-6dof-HandH/scopes/work-in-progress/lab ==
  dYdt : Inport
  Y : Inport  Port=2
  Compare To Constant : simulink/Logic and Bit Operations/Compare To Constant  relop=>=  const=0.0  OutDataTypeStr=boolean
  Demux : Demux  Outputs=[3 3 3 3]
  Demux1 : Demux  Outputs=[3 3 3 3]
  Gain : Gain  Gain=C.RAD2DEG
  Gain1 : Gain  Gain=C.RAD2DEG
  Scope1 : Scope
  Scope9 : Scope
  Selector : Selector  InputPortWidth=3  IndexOptions=Index vector (dialog)  Indices=[3]  OutputSizes=1
  Selector1 : Selector  InputPortWidth=3  IndexOptions=Index vector (dialog)  Indices=[1 2]  OutputSizes=1
  Stop Simulation : Stop
  TH1 : Scope
  TH1dot : Scope
  TH2dot : Scope
  TH2dotdot : Scope
  X1 : Scope
  X1dot : Scope
  X2dot : Scope
  X2dotdot : Scope
  wires:
  Compare To Constant/1 -> Stop Simulation/1
  Selector/1 -> Compare To Constant/1
  Gain/1 -> Scope1/1
  Gain1/1 -> Scope9/1
  Selector1/1 -> TH1/1
  Y/1 -> Demux/1
  Demux/1 -> Selector/1, X1/1
  Demux/2 -> Selector1/1
  Demux/3 -> X2dot/1
  Demux/4 -> TH2dot/1
  dYdt/1 -> Demux1/1
  Demux1/1 -> X1dot/1
  Demux1/2 -> TH1dot/1
  Demux1/4 -> TH2dotdot/1
  Demux1/3 -> X2dotdot/1
  [alpha3] -> Gain/1
  [beta2] -> Gain1/1

== system flatball_6dof/flatball-6dof-HandH/scopes/work-in-progress/side-slip ==
  Y : Inport
  Ground : Ground
  Ground1 : Ground
  Mux : Mux  Inputs=3
  Product : Product  Multiplication=Matrix(*)
  Product1 : Product  Multiplication=Matrix(*)
  TH2dot : Selector  InputPortWidth=12  IndexOptions=Index vector (dialog)  Indices=[10 11 12]  OutputSizes=1
  Transpose : Math  Operator=transpose  SaturateOnIntegerOverflow=on
  X2dot : Selector  InputPortWidth=12  IndexOptions=Index vector (dialog)  Indices=[7 8 9]  OutputSizes=1
  attitude-transformation : MATLAB Function  TreatAsAtomicUnit=on
  X3dot : Outport
  TH3dot : Outport  Port=2
  wires:
  Product1/1 -> TH3dot/1
  Product/1 -> X3dot/1
  TH2dot/1 -> Product1/2  "TH2dot"
  X2dot/1 -> Product/2  "X2dot"
  [Ta23] -> Product1/1, Product/1  "Ta23"
  Y/1 -> TH2dot/1, X2dot/1
  [beta2] -> Mux/3
  Mux/1 -> attitude-transformation/1(TH)
  attitude-transformation/1(T) -> Transpose/1  "Ta32"
  Ground/1 -> Mux/1
  Ground1/1 -> Mux/2
  Transpose/1 -> [Ta23]  "Ta23"

== system flatball_6dof/flatball-6dof-HandH/scopes/work-in-progress/wind-forces-and-moments ==
  CX : Inport
  CTH : Inport  Port=2
  Constant : Constant  Value=amb.rho / 2
  Constant1 : Constant  Value=disc.S
  Constant2 : Constant  Value=disc.c
  Demux : Demux  Outputs=3
  Gain : Gain  Gain=-1
  Gain1 : Gain  Gain=0
  Gain2 : Gain  Gain=-1
  Mux : Mux  Inputs=3
  Product1 : Product  Inputs=3
  Product2 : Product
  Product3 : Product
  Product4 : Product
  Square : Math  Operator=square  SaturateOnIntegerOverflow=on
  F4 : Outport
  M4 : Outport  Port=2
  wires:
  Product1/1 -> M4/1
  Product2/1 -> F4/1
  CTH/1 -> Product1/1
  [qS] -> Product1/2, Product2/2
  CX/1 -> Demux/1
  Demux/1 -> Gain/1
  Demux/2 -> Gain1/1
  Demux/3 -> Gain2/1
  Gain1/1 -> Mux/2
  Gain/1 -> Mux/1
  Gain2/1 -> Mux/3
  Mux/1 -> Product2/1
  Constant1/1 -> Product3/2
  Constant/1 -> Product4/1
  Product4/1 -> Product3/1  "q_inf"
  [v_inf] -> Square/1
  Square/1 -> Product4/2
  Product3/1 -> [qS]
  Constant2/1 -> Product1/3

== system flatball_6dof/flatball-6dof-HandH/calc-F-M/calc-F/aero-coeff/Subsystem ==
  alpha3 : Inport
  1-D Lookup Table : Lookup_n-D  NumberOfTableDimensions=1  BreakpointsForDimension1=disc.aoa_data  Table=disc.Cdrag_data  InterpMethod=Cubic spline  ExtrapMethod=Cubic spline  InternalRulePriority=Speed  RndMeth=Simplest  InputSameDT=on
  Math Function : Math  Operator=square  SaturateOnIntegerOverflow=on
  Product1 : Product  Inputs=**
  Sum1 : Sum
  Sum2 : Sum  Inputs=+-
  Terminator : Terminator
  mg : Constant  Value=disc.CD0
  mg1 : Constant  Value=disc.CDa
  mg2 : Constant  Value=disc.alpha0
  Cdrag : Outport
  wires:
  alpha3/1 -> 1-D Lookup Table/1, Sum2/1
  mg1/1 -> Product1/1
  mg/1 -> Sum1/1
  Product1/1 -> Sum1/2
  Sum2/1 -> Math Function/1
  mg2/1 -> Sum2/2
  Math Function/1 -> Product1/2
  1-D Lookup Table/1 -> Cdrag/1
  Sum1/1 -> Terminator/1

== system flatball_6dof/flatball-6dof-HandH/calc-F-M/calc-F/aero-coeff/Subsystem1 ==
  alpha3 : Inport
  1-D Lookup Table : Lookup_n-D  NumberOfTableDimensions=1  BreakpointsForDimension1=disc.aoa_data  Table=disc.Clift_data  InterpMethod=Cubic spline  ExtrapMethod=Cubic spline  InternalRulePriority=Speed  RndMeth=Simplest  InputSameDT=on
  Product1 : Product  Inputs=**
  Sum1 : Sum
  Terminator : Terminator
  mg : Constant  Value=disc.CL0
  mg1 : Constant  Value=disc.CLa
  Clift : Outport
  wires:
  Product1/1 -> Sum1/2
  mg/1 -> Sum1/1
  mg1/1 -> Product1/1
  alpha3/1 -> 1-D Lookup Table/1, Product1/2
  1-D Lookup Table/1 -> Clift/1
  Sum1/1 -> Terminator/1

== system flatball_6dof/flatball-6dof-HandH/calc-F-M/calc-F/aero-coeff/calc-Cd ==
  alpha : Inport
  Cd0 : Constant  Value=disc.CD0
  Cda : Constant  Value=disc.CDa
  Product : Product
  Square : Math  Operator=square  SaturateOnIntegerOverflow=on
  Sum : Sum  Inputs=+-
  Sum1 : Sum
  alpha0 : Constant  Value=disc.alpha0
  Cd : Outport
  wires:
  Sum1/1 -> Cd/1
  Square/1 -> Product/2
  Product/1 -> Sum1/2
  Cda/1 -> Product/1
  Cd0/1 -> Sum1/1
  Sum/1 -> Square/1
  alpha0/1 -> Sum/2
  alpha/1 -> Sum/1

== system flatball_6dof/flatball-6dof-HandH/calc-F-M/calc-F/aero-coeff/calc-Cl ==
  alpha : Inport
  CL0 : Constant  Value=disc.CL0
  CLa : Constant  Value=disc.CLa
  Product : Product
  Sum1 : Sum
  Cl : Outport
  wires:
  alpha/1 -> Product/2
  CL0/1 -> Sum1/1
  CLa/1 -> Product/1
  Product/1 -> Sum1/2
  Sum1/1 -> Cl/1

== system flatball_6dof/flatball-6dof-HandH/calc-F-M/lab/calc-F/aero-coeff ==
  alpha : Inport
  Subsystem : Subsystem
  Subsystem1 : Subsystem
  Cl : Outport
  Cd : Outport  Port=2
  wires:
  alpha/1 -> Subsystem1/1(alpha), Subsystem/1(alpha)
  Subsystem1/1(Cl) -> Cl/1
  Subsystem/1(Cd) -> Cd/1

== system flatball_6dof/flatball-6dof-HandH/calc-F-M/lab/calc-F/q-inf ==
  X : Inport
  Gain : Gain  Gain=0.5
  Product1 : Product  Inputs=3
  Product2 : Product
  S : Constant  Value=disc.A
  Square : Math  Operator=square  SaturateOnIntegerOverflow=on
  X-to-vel : MATLAB Function  TreatAsAtomicUnit=on
  d : Constant  Value=disc.d
  rho : Constant  Value=amb.rho
  vector-norm : MATLAB Function  TreatAsAtomicUnit=on
  q-inf-S : Outport
  q-inf-S-d : Outport  Port=2
  wires:
  Product1/1 -> Gain/1
  rho/1 -> Product1/3
  X/1 -> X-to-vel/1(X)
  vector-norm/1(norm) -> Square/1
  S/1 -> Product1/2
  Square/1 -> Product1/1
  Gain/1 -> Product2/1, q-inf-S/1
  X-to-vel/1(vel) -> vector-norm/1(vec)
  Product2/1 -> q-inf-S-d/1
  d/1 -> Product2/2

== system flatball_6dof/flatball-6dof-HandH/calc-F-M/lab/calc-M/aero-coeff ==
  alpha : Inport
  Subsystem2 : Subsystem
  Cm : Outport
  wires:
  alpha/1 -> Subsystem2/1(alpha)
  Subsystem2/1(Cm) -> Cm/1
